simulink model "tempppp"  (R2020b)
settings: Solver=VariableStepAuto  StartTime=0.0  StopTime=10.0  RelTol=1e-3
settings Model: Creator=Jonathan van Zyl  LastModifiedBy=Jonathan van Zyl

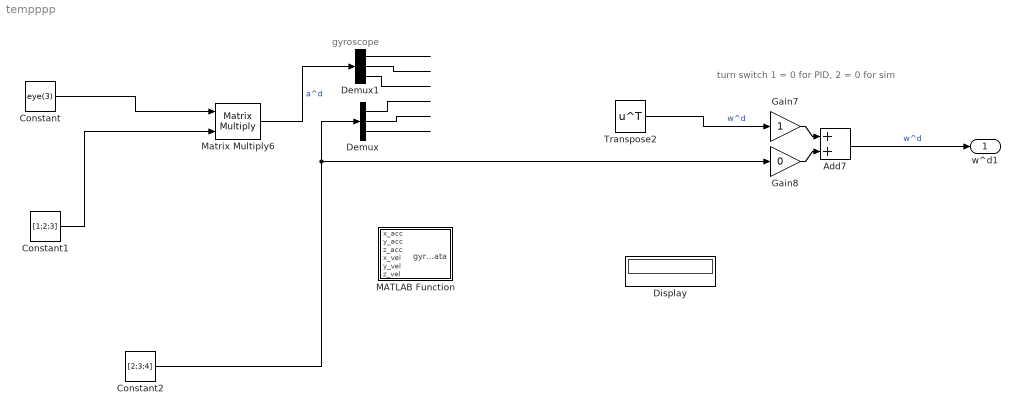
== system tempppp ==
  note: turn switch 1 = 0 for PID, 2 = 0 for sim
  note: gyroscope
  Add7 : Sum
  Constant : Constant  Value=eye(3)  VectorParams1D=off
  Constant1 : Constant  Value=[1;2;3]  VectorParams1D=off
  Constant2 : Constant  Value=[2;3;4]  VectorParams1D=off
  Demux : Demux  Outputs=3
  Demux1 : Demux  Outputs=3
  Display : Display
  Gain7 : Gain
  Gain8 : Gain  Gain=0
  MATLAB Function : MATLAB Function  TreatAsAtomicUnit=on
  Matrix Multiply6 : Product  Multiplication=Matrix(*)
  Transpose2 : Math  Operator=transpose  SaturateOnIntegerOverflow=on
  w^d1 : Outport
  wires:
  Constant2/1 -> Gain8/1, Demux/1
  Matrix Multiply6/1 -> Demux1/1  "a^d"
  Demux/3 -> ?
  Demux1/3 -> ?
  Add7/1 -> w^d1/1  "w^d"
  Demux/2 -> ?
  Demux1/2 -> ?
  Gain8/1 -> Add7/2
  Transpose2/1 -> Gain7/1  "w^d"
  Demux1/1 -> ?
  Gain7/1 -> Add7/1
  Constant1/1 -> Matrix Multiply6/2
  ? -> Display/1, Transpose2/1  "w^d_sensed"
  Demux/1 -> ?
  Constant/1 -> Matrix Multiply6/1

== matlab function tempppp/MATLAB Function ==
  data: x_acc input; gyroData output; y_acc input; z_acc input; x_vel input; y_vel input; z_vel input
function gyroData  = gyroscope(x_acc, y_acc, z_acc, x_vel, y_vel, z_vel)
    % Ouputs: Angular velocity
    % Create gyroscope sensor object
    acc = [x_acc, y_acc, z_acc];
    angvel = [x_vel, y_vel, z_vel];
    
    params = gyroparams;         
    
    % Parameters for simulated signal
    N = 1;       % Number of samples
    Fs = 100;       % Sampling rate
    Fc = 0.25;      % Sinusoidal frequency
    
    % Create arrays
    t = (0:(1/Fs):((N-1)/Fs)).';
    acc = acc;          % Input accelerations
    angvel = angvel;
    %angvel(:,1) = 8*sin(2*pi*Fc*t);
    
    % Generate gyroscopic data
    imu = imuSensor('SampleRate', Fs, 'Gyroscope', params);
    imu.Gyroscope.MeasurementRange = 6.5;   % Maximum angular velocity gyroscope can measure
    imu.Gyroscope.Resolution = 1/Fs;           % Step size of digital measurements
    
    % Biases
    
    imu.Gyroscope.BiasInstability = 0.12 * 3.14159 / 180;       % rad/hr
    imu.Gyroscope.NoiseDensity = 0.15 * 3.14159 / 180;          % rad/s
    imu.Gyroscope.RandomWalk = 0.017 * 3.14159 / 180;           % rad/sqrt(hr)
    imu.Gyroscope.TemperatureBias = 0.25 * 3.14159 / 180;       % rad/s
    %imu.Gyroscope.AccelerationBias = 0.3;
    
    % Define real accelerations
    %acc(:,1) = 1;
    [~, gyroData] = imu(acc, angvel);

end
